simulink model "test_car_2021"  (R2021b)
settings: Solver=ode45  StartTime=0.0  StopTime=120  RelTol=1e-3
model workspace (MAT data in the model file):
  Ah = 5200
  J = 0.01
  K = 0.01
  L = 0.01
  R = 0.01
  af = 0.57
  b = 0.1
  c1 = 2e-06
  cdrag = 0.37
  k0 = 380
  k2 = 2
  k3 = 20
  k4 = -5
  mass = 300
  rho = 1.18
  socInit = 1
  vnom = 400
  wheelRadius = 0.3
settings Model: Creator=sansh  LastModifiedBy=mg2124
settings SolverCC: AlgebraicLoopSolver=TrustRegion
settings DataIOCC: ReturnWorkspaceOutputs=off
settings DebuggingCC: SFMachineParentedDataDiag=warning  ArithmeticOperatorsInVariantConditions=warning
settings SFSimCC: SimUseLocalCustomCode=off  CustomCodeUndefinedFunction=UseInterfaceOnly
settings RTWCC: RTWUseLocalCustomCode=off  DLArmComputeVersion=20.02.1
settings CodeAppCC: StateflowObjectComments=on

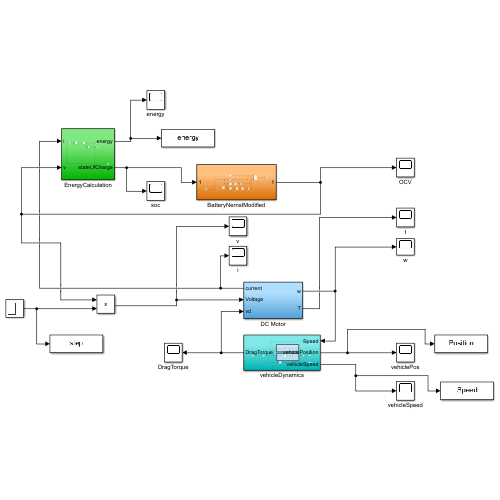
[thumbnail: Simulink's stored preview of the top-level diagram]
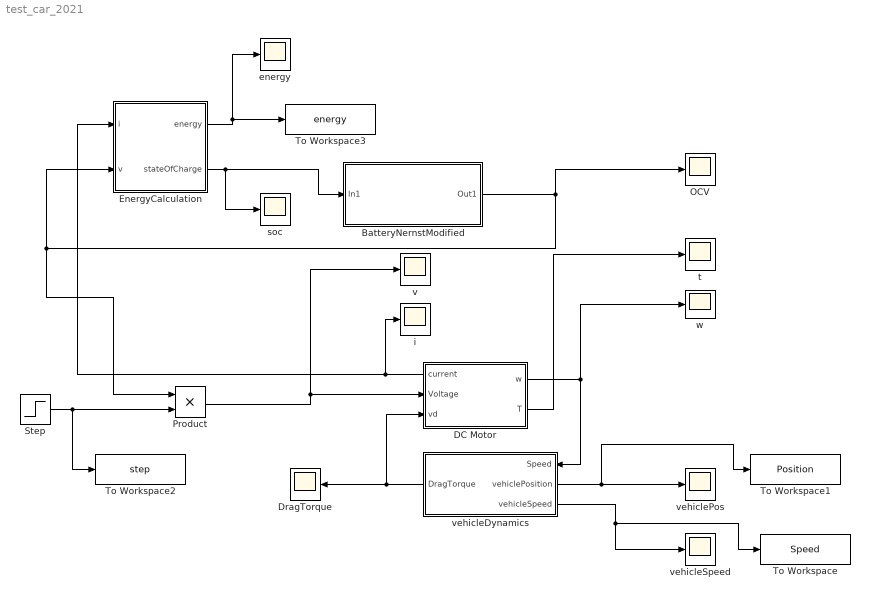
== system test_car_2021 ==
  BatteryNernstModified : Subsystem
  DC Motor : Subsystem
      settings: PortSchema="{\"entries\":[{\"content\":{\"sides\":[{\"content\":{\"connectorIds\":[\"Out3\",\"In1\",\"In2\"]},\"type\":\"ConnectorPlacement.EquallySpacedRectSide\",\"uuid\":\"b276cc4c-6e56-4956-8f44-003124433d7e\"},{\"content\":{\"connectorIds\":[\"Out1\",\"Out2\"],\"side\":\"RIGHT\"},\"type\":\"ConnectorPlacement.EquallySpacedRectSide\",\"uuid\":\"98d555dc-4bec-4179-83d1-7f47ef529afe\"},{\"content\":{\"connectorIds\":[],\"side\":\"TOP\"},\"type\":\"ConnectorPlacement.EquallySpacedRectSide\",\"uuid\":\"179053d8-aed3-445b-8bde-cf864afeeb53\"}]},\"type\":\"ConnectorPlacement.EquallySpacedConnector\",\"uuid\":\"b402df6a-fe5a-46c9-a6de-67aaf8332b13\"}],\"packageUris\":[\"http://schema.mathworks.com/mf0/Connector/R2020b\"],\"version\":\"1.0\"}"
  DragTorque : Scope
  EnergyCalculation : Subsystem
  OCV : Scope
  Product : Product
  Step : Step  Before=1  SampleTime=0
  To Workspace : ToWorkspace  VariableName=Speed  SampleTime=-1
  To Workspace1 : ToWorkspace  VariableName=Position  SampleTime=-1
  To Workspace2 : ToWorkspace  VariableName=step  SampleTime=-1
  To Workspace3 : ToWorkspace  VariableName=energy  SampleTime=-1
  energy : Scope
  i : Scope
  soc : Scope
  t : Scope
  v : Scope
  vehicleDynamics : Subsystem
      settings: PortSchema="{\"entries\":[{\"content\":{\"sides\":[{\"content\":{\"connectorIds\":[\"In1\",\"Out2\",\"Out3\"]},\"type\":\"ConnectorPlacement.EquallySpacedRectSide\",\"uuid\":\"07ecf1cb-0d5c-4608-88cc-e61117b79db0\"},{\"content\":{\"connectorIds\":[\"Out1\"],\"side\":\"RIGHT\"},\"type\":\"ConnectorPlacement.EquallySpacedRectSide\",\"uuid\":\"003f7a32-9b2b-44d7-acb6-981f8f38bf0d\"},{\"content\":{\"connectorIds\":[],\"side\":\"TOP\"},\"type\":\"ConnectorPlacement.EquallySpacedRectSide\",\"uuid\":\"864d97b5-3a75-4ab5-b9c0-20b3f38956ab\"}]},\"type\":\"ConnectorPlacement.EquallySpacedConnector\",\"uuid\":\"7c02dec8-5acc-4a8e-8ac6-d1d16052955e\"}],\"packageUris\":[\"http://schema.mathworks.com/mf0/Connector/R2020b\"],\"version\":\"1.0\"}"
  vehiclePos : Scope
  vehicleSpeed : Scope
  w : Scope
  wires:
  DC Motor/1(w) -> vehicleDynamics/1(Speed), w/1
  DC Motor/3(current) -> EnergyCalculation/1(i), i/1
  DC Motor/2(T) -> t/1
  vehicleDynamics/1(DragTorque) -> DC Motor/2(vd), DragTorque/1
  vehicleDynamics/2(vehiclePosition) -> To Workspace1/1, vehiclePos/1
  vehicleDynamics/3(vehicleSpeed) -> vehicleSpeed/1, To Workspace/1
  EnergyCalculation/1(energy) -> To Workspace3/1, energy/1
  EnergyCalculation/2(stateOfCharge) -> BatteryNernstModified/1(In1), soc/1
  Step/1 -> To Workspace2/1, Product/2
  Product/1 -> v/1, DC Motor/1(Voltage)
  BatteryNernstModified/1(Out1) -> OCV/1, EnergyCalculation/2(v), Product/1

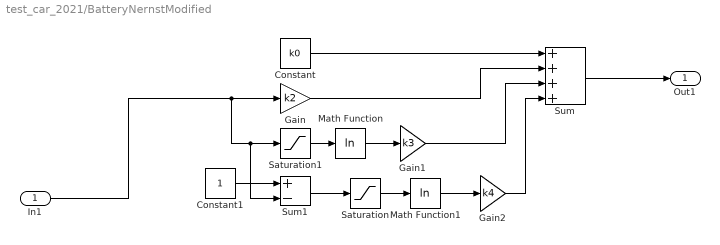
== system test_car_2021/BatteryNernstModified ==
  In1 : Inport
  Constant : Constant  Value=k0
  Constant1 : Constant
  Gain : Gain  Gain=k2
  Gain1 : Gain  Gain=k3
  Gain2 : Gain  Gain=k4
  Math Function : Math  Operator=log  SaturateOnIntegerOverflow=on
  Math Function1 : Math  Operator=log  SaturateOnIntegerOverflow=on
  Saturation : Saturate  UpperLimit=1  LowerLimit=0.01
  Saturation1 : Saturate  UpperLimit=1  LowerLimit=0.01
  Sum : Sum  Inputs=++++
  Sum1 : Sum  Inputs=+-
  Out1 : Outport
  wires:
  Gain2/1 -> Sum/4
  Sum1/1 -> Saturation/1
  Saturation/1 -> Math Function1/1
  Constant/1 -> Sum/1
  Math Function1/1 -> Gain2/1
  Math Function/1 -> Gain1/1
  Constant1/1 -> Sum1/1
  Gain1/1 -> Sum/3
  Saturation1/1 -> Math Function/1
  Sum/1 -> Out1/1
  Gain/1 -> Sum/2
  In1/1 -> Saturation1/1, Sum1/2, Gain/1

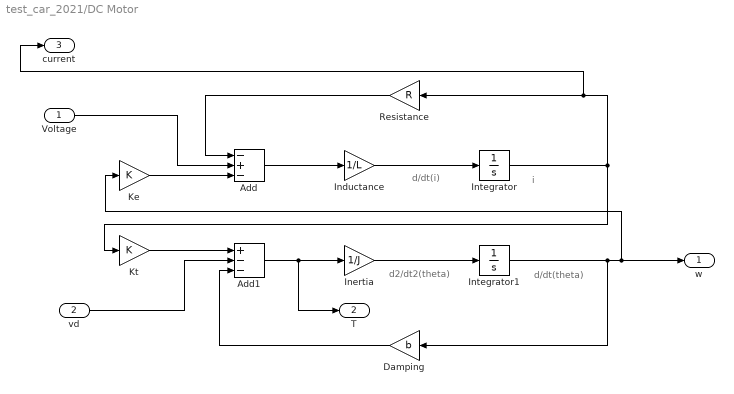
== system test_car_2021/DC Motor ==
  note: i
  note: d/dt(i)
  note: d/dt(theta)
  note: d2/dt2(theta)
  Voltage : Inport
  vd : Inport  Port=2
  Add : Sum  Inputs=-+-
  Add1 : Sum  Inputs=+--
  Damping : Gain  Gain=b
  Inductance : Gain  Gain=1/L
  Inertia : Gain  Gain=1/J
  Integrator : Integrator
  Integrator1 : Integrator
  Ke : Gain  Gain=K
  Kt : Gain  Gain=K
  Resistance : Gain  Gain=R
  w : Outport
  T : Outport  Port=2
  current : Outport  Port=3
  wires:
  Inductance/1 -> Integrator/1
  Integrator1/1 -> Damping/1, w/1, Ke/1
  Inertia/1 -> Integrator1/1
  Integrator/1 -> current/1, Resistance/1, Kt/1
  Kt/1 -> Add1/1
  Voltage/1 -> Add/2
  Resistance/1 -> Add/1
  Damping/1 -> Add1/3
  Ke/1 -> Add/3
  Add/1 -> Inductance/1
  Add1/1 -> T/1, Inertia/1
  vd/1 -> Add1/2

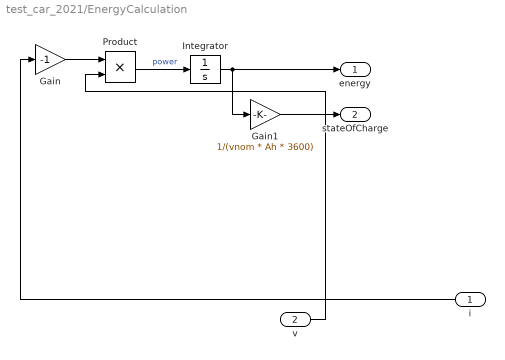
== system test_car_2021/EnergyCalculation ==
  i : Inport
  v : Inport  Port=2
  Gain : Gain  Gain=-1
  Gain1 : Gain  Gain=1/(vnom * Ah * 3600)
  Integrator : Integrator  InitialCondition=socInit * vnom * Ah * 3600
  Product : Product
  energy : Outport
  stateOfCharge : Outport  Port=2
  wires:
  v/1 -> Product/2
  i/1 -> Gain/1
  Product/1 -> Integrator/1  "power"
  Gain1/1 -> stateOfCharge/1
  Gain/1 -> Product/1
  Integrator/1 -> energy/1, Gain1/1

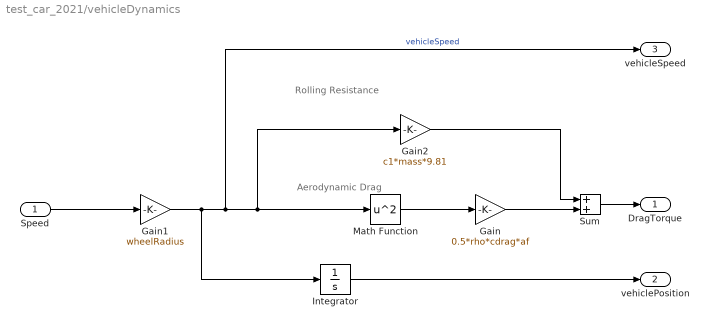
== system test_car_2021/vehicleDynamics ==
  note: Rolling Resistance
  note: Aerodynamic Drag
  Speed : Inport
  Gain : Gain  Gain=0.5*rho*cdrag*af
  Gain1 : Gain  Gain=wheelRadius
  Gain2 : Gain  Gain=c1*mass*9.81
  Integrator : Integrator
  Math Function : Math  Operator=square  SaturateOnIntegerOverflow=on
  Sum : Sum
  DragTorque : Outport
  vehiclePosition : Outport  Port=2
  vehicleSpeed : Outport  Port=3
  wires:
  Gain/1 -> Sum/2
  Speed/1 -> Gain1/1
  Math Function/1 -> Gain/1
  Gain1/1 -> Gain2/1, Math Function/1, vehicleSpeed/1, Integrator/1  "vehicleSpeed"
  Integrator/1 -> vehiclePosition/1
  Sum/1 -> DragTorque/1
  Gain2/1 -> Sum/1
